simulink model "prob2"  (R2020b)
settings: Solver=VariableStepAuto  StartTime=0.0  StopTime=10  RelTol=1e-3
settings Model: Creator=Nitin  LastModifiedBy=Nitin

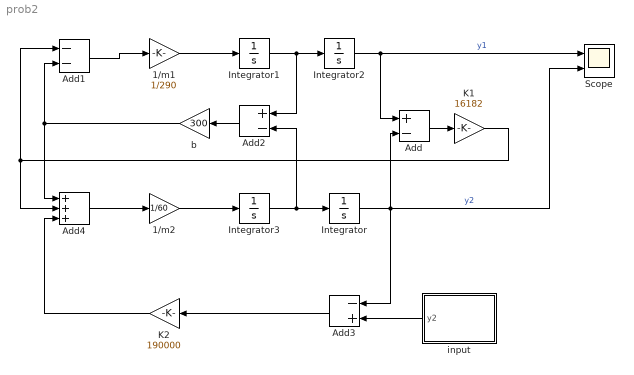
== system prob2 ==
  1/m1 : Gain  Gain=1/290
  1/m2 : Gain  Gain=1/60
  Add : Sum  Inputs=+-
  Add1 : Sum  Inputs=--
  Add2 : Sum  Inputs=+-
  Add3 : Sum  Inputs=-+
  Add4 : Sum  Inputs=+++
  Integrator{,1..3} (4 alike) : Integrator
  K1 : Gain  Gain=16182
  K2 : Gain  Gain=190000
  Scope : Scope  NumInputPorts=2
  b : Gain  Gain=300
  input : MATLAB Function  TreatAsAtomicUnit=on
  wires:
  1/m1/1 -> Integrator1/1
  Integrator3/1 -> Add2/2, Integrator/1
  Integrator/1 -> Add3/1, Add/2, Scope/2  "y2"
  Integrator2/1 -> Add/1, Scope/1  "y1"
  Add3/1 -> K2/1
  Add/1 -> K1/1
  Integrator1/1 -> Add2/1, Integrator2/1
  Add2/1 -> b/1
  Add1/1 -> 1/m1/1
  Add4/1 -> 1/m2/1
  1/m2/1 -> Integrator3/1
  b/1 -> Add4/1, Add1/2
  K2/1 -> Add4/3
  K1/1 -> Add4/2, Add1/1
  input/1(y2) -> Add3/2

== matlab function prob2/input ==
  data: y2 output
function y2 = fcn

t=linspace(0,100);
y=sin(t);
y(t>pi)=0;

y2=round(y)
hold on
plot(y2,'b')
xlabel("Time(sec)")
ylabel("Amplitude")
title("dummy signal")
